simulink model "SF045A_HwAgSysArbn"  (R2013b)
settings: Solver=FixedStepDiscrete  SolverMode=SingleTasking  StartTime=0.0  StopTime=1  FixedStep=.002  RelTol=1e-3
values from neighbouring files (symbols this model uses):
  ARCHGLBPRM_2MILLISEC_SEC_F32 = DataDict.Constant    [SF045A_HwAgSysArbn_DataDict.m]
  ARCHGLBPRM_FLOATZEROTHD_ULS_F32 = DataDict.Constant    [SF045A_HwAgSysArbn_DataDict.m]
  ARCHGLBPRM_PIOVER180_ULS_F32 = DataDict.Constant    [SF045A_HwAgSysArbn_DataDict.m]
  CNVSECTOCNT_ULS_U32 = DataDict.Constant    [SF045A_HwAgSysArbn_DataDict.m]
  CNVTOMILLISEC_MILLISECPERCNT_F32 = DataDict.Constant    [SF045A_HwAgSysArbn_DataDict.m]
  FltInj_f32 = DataDict.Client    [SF045A_HwAgSysArbn_DataDict.m]
  FLTINJ_HWAGSYSARBN_HWAG = DataDict.Constant    [SF045A_HwAgSysArbn_DataDict.m]
  FLTINJ_HWAGSYSARBN_SERLCOMHWAG = DataDict.Constant    [SF045A_HwAgSysArbn_DataDict.m]
  HwAgCorrlnFlt = DataDict.NTC    [SF045A_HwAgSysArbn_DataDict.m]
  HwAgSnsrlsThdExcdd = DataDict.NTC    [SF045A_HwAgSysArbn_DataDict.m]
  HwAgSysArbnHwAgConf1Snsr = DataDict.Calibration    [SF045A_HwAgSysArbn_DataDict.m]
  HwAgSysArbnHwAgConf2Snsr = DataDict.Calibration    [SF045A_HwAgSysArbn_DataDict.m]
  HwAgSysArbnHwAgConfNoSnsr = DataDict.Calibration    [SF045A_HwAgSysArbn_DataDict.m]
  HwAgSysArbnHwAgCorrdCorrlnThd = DataDict.Calibration    [SF045A_HwAgSysArbn_DataDict.m]
  HwAgSysArbnHwAgCorrlnFailDebStep = DataDict.Calibration    [SF045A_HwAgSysArbn_DataDict.m]
  HwAgSysArbnHwAgCorrlnPassDebStep = DataDict.Calibration    [SF045A_HwAgSysArbn_DataDict.m]
  HwAgSysArbnHwAgCorrlnRng = DataDict.Calibration    [SF045A_HwAgSysArbn_DataDict.m]
  HwAgSysArbnHwAgSlewRate = DataDict.Calibration    [SF045A_HwAgSysArbn_DataDict.m]
  HwAgSysArbnHwAgSnsrlsCorrlnThd = DataDict.Calibration    [SF045A_HwAgSysArbn_DataDict.m]
  HwAgSysArbnHwAgSnsrlsKineThd = DataDict.Calibration    [SF045A_HwAgSysArbn_DataDict.m]
  HwAgSysArbnHwAgToMotAgCorrlnElpdTiLim = DataDict.Calibration    [SF045A_HwAgSysArbn_DataDict.m]
  HwAgSysArbnSerlComHwAgCorrdConf = DataDict.Calibration    [SF045A_HwAgSysArbn_DataDict.m]
  HwAgSysArbnSerlComHwAgSnsrlsConf = DataDict.Calibration    [SF045A_HwAgSysArbn_DataDict.m]
  HwAgSysArbnSlewRateTmr = DataDict.Calibration    [SF045A_HwAgSysArbn_DataDict.m]
  HWAGTHD_ULS_FLOAT32 = DataDict.Constant    [SF045A_HwAgSysArbn_DataDict.m]
  INVLDSRC_CNT_S08 = DataDict.Constant    [SF045A_HwAgSysArbn_DataDict.m]
  LRGSLEW_HWDEGPERSEC_F32 = DataDict.Constant    [SF045A_HwAgSysArbn_DataDict.m]
  NODEBSTEP_CNT_U16 = DataDict.Constant    [SF045A_HwAgSysArbn_DataDict.m]
  SLEWINPROGS_CNT_LGC = DataDict.Constant    [SF045A_HwAgSysArbn_DataDict.m]
  SLEWNOTINPROGS_CNT_LGC = DataDict.Constant    [SF045A_HwAgSysArbn_DataDict.m]
  SNSRDATASRCSELD_CNT_S08 = DataDict.Constant    [SF045A_HwAgSysArbn_DataDict.m]
  SNSRLSDATASRCSELD_CNT_S08 = DataDict.Constant    [SF045A_HwAgSysArbn_DataDict.m]
  SysGlbPrmSysKineRat = DataDict.ImprtdCal    [SF045A_HwAgSysArbn_DataDict.m]
  SysGlbPrmTorsBarStfn = DataDict.ImprtdCal    [SF045A_HwAgSysArbn_DataDict.m]
  ZEROTMR_MILLISEC_F32 = DataDict.Constant    [SF045A_HwAgSysArbn_DataDict.m]
undefined symbols (not defined in the file or in its folder): NtcSts1
libraries: NxtrLim x11, simulink x6, NxtrAbslt x6, Fil x3, autosarlib x2
(part 2 of 6)

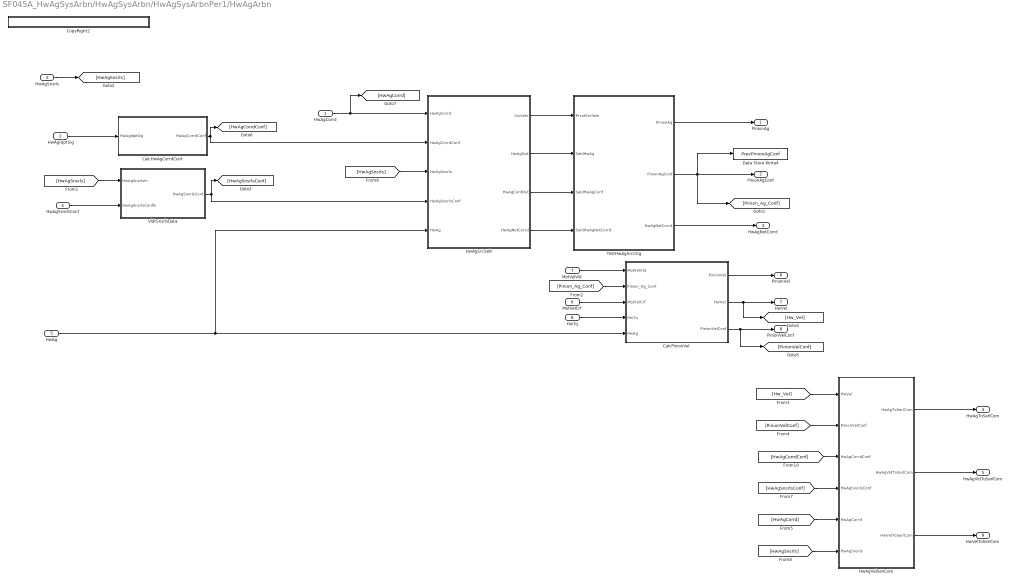
== system SF045A_HwAgSysArbn/HwAgSysArbn/HwAgSysArbnPer1/HwAgArbn ==
  HwAgCorrd : Inport
  HwAgIdptSig : Inport  Port=2
  HwAgSnsrls : Inport  Port=3
  HwAgSnsrlsConf : Inport  Port=4
  HwAg : Inport  Port=5
  MotVelCrf : Inport  Port=6
  MotVelVld : Inport  Port=7
  HwTq : Inport  Port=8
  "CalcHwAgCorrdConf " : Subsystem  RequirementInfo="{'linktype_rmi_doors' '00012ce0 (/E-STEER Core/SubSystem Specifications/Application Functions - EA4/SF045A Handwheel Angle System Arbitration)' '#SF045A_68' 'true' 'REQ:  SF045A_68' '' } %GIDa_6372da7c_5ece_4f0a_8ac6_d737184b35a8"
  CalcPinionVel : Subsystem  RequirementInfo="{'linktype_rmi_doors' '00012ce0 (/E-STEER Core/SubSystem Specifications/Application Functions - EA4/SF045A Handwheel Angle System Arbitration)' '#SF045A_138' 'true' 'REQ:  SF045A_138' '' ; 'linktype_rmi_doors' '00012ce0 (/E-STEER Core/SubSystem Specifications/Application Functions - EA4/SF045A Handwheel Angle System Arbitration)' '#SF045A_139' 'true' 'REQ:  SF045A_139' '' ; 'linktype_rmi_doors' '00012ce0 (/E-STEER Core/SubSystem Specifications/Application Functions - EA4/SF045A Handwheel Angle System Arbitration)' '#SF045A_140' 'true' 'REQ:  SF045A_140' '' ; 'linktype_rmi_doors' '00012ce0 (/E-STEER Core/SubSystem Specifications/Application Functions - EA4/SF045A Handwheel Angle System Arbitration)' '#SF045A_137' 'true' 'REQ:  SF045A_137' '' } %GIDa_9cefdf0b_14fb_482a_9d83_2c4a3ede8765"
  CopyRight2 : Subsystem  Description=|  mask(Copyright Information){none=on}
      | Copyright info block.                                               
      |                                                                     
      | Place copyright information at the top of every subsystem in design.
      mask prompts: none "No parameters"
      mask help: Place copyright information at the top of every subsystem in design.
      mask Display:
      | NxtrConf = 'Nexteer Confidential';
      | 
      | sys = bdroot; %handle for the current model ("system")
      | first = get_param(sys,'Created');
      | first = first(end-3:end);  %year is last four digits
      | 
      | last = get_param(sys,'LastModifiedDate');
      | if isempty(last)
      |     last = datestr(now,'yyyy');
      | else
      |     last = last(end-3:end);
      | end
      | 
      | if strcmp(first,last)
      |     fprintf('%s -- Copyright %s Nexteer',NxtrConf,first)
      | else
      |     fprintf('%s -- %s%s- %s Nexteer',NxtrConf,char(169),first,last)
      | end
  Data Store Write4 : DataStoreWrite  RequirementInfo={} %GIDa_c1ebf7a9_2516_4ce7_952f_4fdc50b92ec1  DataStoreName=PrevPinionAgConf
  HwAgSrcSeln : Subsystem  RequirementInfo="{'linktype_rmi_doors' '00012ce0 (/E-STEER Core/SubSystem Specifications/Application Functions - EA4/SF045A Handwheel Angle System Arbitration)' '#SF045A_71' 'true' 'REQ:  SF045A_71' '' } %GIDa_ddb011fd_98f7_44d7_8620_c4b3bd53cfc5"
  HwAgVelSeriCom : Subsystem  RequirementInfo="{'linktype_rmi_doors' '00012ce0 (/E-STEER Core/SubSystem Specifications/Application Functions - EA4/SF045A Handwheel Angle System Arbitration)' '#SF045A_85' 'true' 'REQ:  SF045A_85' '' ; 'linktype_rmi_doors' '00012ce0 (/E-STEER Core/SubSystem Specifications/Application Functions - EA4/SF045A Handwheel Angle System Arbitration)' '#SF045A_86' 'true' 'REQ:  SF045A_86' '' ; 'linktype_rmi_doors' '00012ce0 (/E-STEER Core/SubSystem Specifications/Application Functions - EA4/SF045A Handwheel Angle System Arbitration)' '#SF045A_141' 'true' 'REQ:  SF045A_141' '' ; 'linktype_rmi_doors' '00012ce0 (/E-STEER Core/SubSystem Specifications/Application Functions - EA4/SF045A Handwheel Angle System Arbitration)' '#SF045A_90' 'true' 'REQ:  SF045A_90' '' ; 'linktype_rmi_doors' '00012ce0 (/E-STEER Core/SubSystem Specifications/Application Functions - EA4/SF045A Handwheel Angle System Arbitration)' '#SF045A_87' 'true' 'REQ:  SF045A_87' '' ; 'linktype_rmi_doors' '00012ce0 (/E-STEER Core/SubSystem Specifications/Application Functions - EA4/SF045A Handwheel Angle System Arbitration)' '#SF045A_126' 'true' 'REQ:  SF045A_126' '' ; 'linktype_rmi_doors' '00012ce0 (/E-STEER Core/SubSystem Specifications/Application Functions - EA4/SF045A Handwheel Angle System Arbitration)' '#SF045A_124' 'true' 'REQ:  SF045A_124' '' ; 'linktype_rmi_doors' '00012ce0 (/E-STEER Core/SubSystem Specifications/Application Functions - EA4/SF045A Handwheel Angle System Arbitration)' '#SF045A_88' 'true' 'REQ:  SF045A_88' '' } %GIDa_7881f2ec_efdf_43f2_b299_16eeb03e4f64"
  TestHwAgSrcChg : Subsystem
  VldtSnsrlsData : Subsystem  RequirementInfo="{'linktype_rmi_doors' '00012ce0 (/E-STEER Core/SubSystem Specifications/Application Functions - EA4/SF045A Handwheel Angle System Arbitration)' '#SF045A_69' 'true' 'REQ:  SF045A_69' '' } %GIDa_369b4bc0_9330_46ed_81c8_e018ed0a07fe"
  PinionAg : Outport
  PinionAgConf : Outport  Port=2
  HwAgNotCorrd : Outport  Port=3
  HwAgToSerlCom : Outport  Port=4
  HwAgVldToSerlCom : Outport  Port=5
  PinionVel : Outport  Port=6
  HwVel : Outport  Port=7
  PinionVelConf : Outport  Port=8
  HwVelToSerlCom : Outport  Port=9
  wires:
  HwAgSrcSeln/1(SrcSeln) -> TestHwAgSrcChg/1(PrsntSrcSeln)
  HwAgSrcSeln/2(HwAgOut) -> TestHwAgSrcChg/2(SeldHwAg)
  HwAgSrcSeln/3(HwAgConfOut) -> TestHwAgSrcChg/3(SeldHwAgConf)
  HwAgSrcSeln/4(HwAgNotCorrd) -> TestHwAgSrcChg/4(SeldHwAgNotCorrd)
  TestHwAgSrcChg/1(PinionAg) -> PinionAg/1
  TestHwAgSrcChg/3(HwAgNotCorrd) -> HwAgNotCorrd/1
  [HwAgSnsrls] -> HwAgSrcSeln/3(HwAgSnsrls)
  HwAgSnsrlsConf/1 -> VldtSnsrlsData/2(HwAgSnsrlsConfIn)
  HwAgSnsrls/1 -> [HwAgSnsrls]
  HwAgCorrd/1 -> [HwAgCorrd], HwAgSrcSeln/1(HwAgCorrd)
  VldtSnsrlsData/1(HwAgSnsrlsConf) -> [HwAgSnsrlsConf], HwAgSrcSeln/4(HwAgSnsrlsConf)
  HwAgIdptSig/1 -> "CalcHwAgCorrdConf "/1(HwAgIdptSig)
  "CalcHwAgCorrdConf "/1(HwAgCorrdConf) -> [HwAgCorrdConf], HwAgSrcSeln/2(HwAgCorrdConf)
  HwAgVelSeriCom/1(HwAgToSerlCom) -> HwAgToSerlCom/1
  HwAgVelSeriCom/2(HwAgVldToSerlCom) -> HwAgVldToSerlCom/1
  [HwAgSnsrls] -> VldtSnsrlsData/1(HwAgSnsrlsIn)
  TestHwAgSrcChg/2(PinionAgConf) -> Data Store Write4/1, [Pinion_Ag_Conf], PinionAgConf/1
  MotVelCrf/1 -> CalcPinionVel/3(MotVelCrf)
  MotVelVld/1 -> CalcPinionVel/1(MotVelVld)
  HwTq/1 -> CalcPinionVel/4(HwTq)
  CalcPinionVel/1(PinionVel) -> PinionVel/1
  CalcPinionVel/2(HwVel) -> [Hw_Vel], HwVel/1
  CalcPinionVel/3(PinionVelConf) -> [PinionVelConf], PinionVelConf/1
  HwAg/1 -> HwAgSrcSeln/5(HwAg), CalcPinionVel/5(HwAg)
  HwAgVelSeriCom/3(HwVelToSerlCom) -> HwVelToSerlCom/1
  [Hw_Vel] -> HwAgVelSeriCom/1(HwVel)
  [PinionVelConf] -> HwAgVelSeriCom/2(PinionVelConf)
  [HwAgCorrdConf] -> HwAgVelSeriCom/3(HwAgCorrdConf)
  [HwAgSnsrlsConf] -> HwAgVelSeriCom/4(HwAgSnsrlsConf)
  [Pinion_Ag_Conf] -> CalcPinionVel/2(Pinion_Ag_Conf)
  [HwAgCorrd] -> HwAgVelSeriCom/5(HwAgCorrd)
  [HwAgSnsrls] -> HwAgVelSeriCom/6(HwAgSnsrls)

== system SF045A_HwAgSysArbn/HwAgSysArbn/HwAgSysArbnInit1/GetRefTmr100MicroSec32bit/CopyRight2 ==

== system SF045A_HwAgSysArbn/HwAgSysArbn/HwAgSysArbnInit1/Kinematic Integrity/SetNtcSts ==
  note: Note:
      |
      | - "ISO Fault Debounce Design" Simulink block intent to use here for Simulation purpose only. Do not Code this block
  NtcNr : Inport
  NtcStInfo : Inport  Port=2
  NtcSts : Inport  Port=3
  DebStep : Inport  Port=4
  CopyRight2 : Subsystem  Description=|  mask(Copyright Information){none=on}
      | Copyright info block.                                               
      |                                                                     
      | Place copyright information at the top of every subsystem in design.
      mask prompts: none "No parameters"
      mask help: Place copyright information at the top of every subsystem in design.
      mask Display:
      | NxtrConf = 'Nexteer Confidential';
      | 
      | sys = bdroot; %handle for the current model ("system")
      | first = get_param(sys,'Created');
      | if(isempty(first))
      |     first = datestr(now,'yyyy');
      | else
      |     first = first(end-3:end);  %year is last four digits
      | end
      | 
      | last = get_param(sys,'LastModifiedDate');
      | if isempty(last)
      |     last = datestr(now,'yyyy');
      | else
      |     last = last(end-3:end);
      | end
      | 
      | if strcmp(first,last)
      |     fprintf('%s -- Copyright %s Nexteer',NxtrConf,first)
      | else
      |     fprintf('%s -- %s%s- %s Nexteer',NxtrConf,char(169),first,last)
      | end
  Data Store Write : DataStoreWrite  DataStoreName=NtcQlfr
  Data Store Write1 : DataStoreWrite  DataStoreName=NtcQlfrHwAgSnsrlsThdExcd
  Data Store Write2 : DataStoreWrite  DataStoreName=NtcStInfoHwAgSnsrlsThdExcd
  Data Store Write3 : DataStoreWrite  DataStoreName=NtcStsHwAgSnsrlsThdExcd
  Data Type Conversion : DataTypeConversion  OutDataTypeStr=Enum: SigQlfr1
  Data Type Conversion1 : DataTypeConversion  OutDataTypeStr=uint8
  Ground : Ground
  ISO Fault Debounce Design : Stateflow chart  TreatAsAtomicUnit=on
      settings: AttributesFormatString=|
      | Simulation Purpose Only.
      | Do Not Code this block
      | Diagnostic Manager Owns this requirement
  Terminator : Terminator
  Terminator1 : Terminator
  wires:
  Data Type Conversion1/1 -> Data Store Write2/1
  NtcStInfo/1 -> Terminator1/1, Data Type Conversion1/1
  NtcSts/1 -> ISO Fault Debounce Design/1(NtcSts), Data Store Write3/1
  Data Type Conversion/1 -> Data Store Write/1, Data Store Write1/1
  Ground/1 -> ISO Fault Debounce Design/3(SvcClr)
  ISO Fault Debounce Design/1(Qualifier) -> Data Type Conversion/1
  DebStep/1 -> ISO Fault Debounce Design/2(DebStep)
  NtcNr/1 -> Terminator/1

== system SF045A_HwAgSysArbn/HwAgSysArbn/HwAgSysArbnPer1/FltInj_f32 client/CodeGen ==
  note: FltInj_f32(float32 *SigPah, uint16 LocnKey)
  note: NOTE 1:  Simulink 2013b cannot handle InOut arguments, so the operation
      |                 prototype inside this block is not quite right.
      |
      | NOTE 2:  Do not use this variant for simulation.  Sig_Out = zero, always.
  Sig : Inport
  "LocnKey  " : Inport  Port=2
  CopyRight1 : Subsystem  Description=|  mask(Copyright Information){none=on}
      | Copyright info block.                                               
      |                                                                     
      | Place copyright information at the top of every subsystem in design.
      mask prompts: none "No parameters"
      mask help: Place copyright information at the top of every subsystem in design.
      mask Display:
      | NxtrConf = 'Nexteer Confidential';
      | 
      | sys = bdroot; %handle for the current model ("system")
      | first = get_param(sys,'Created');
      | if(isempty(first))
      |     first = datestr(now,'yyyy');
      | else
      |     first = first(end-3:end);  %year is last four digits
      | end
      | 
      | last = get_param(sys,'LastModifiedDate');
      | if isempty(last)
      |     last = datestr(now,'yyyy');
      | else
      |     last = last(end-3:end);
      | end
      | 
      | if strcmp(first,last)
      |     fprintf('%s -- Copyright %s Nexteer',NxtrConf,first)
      | else
      |     fprintf('%s -- %s%s- %s Nexteer',NxtrConf,char(169),first,last)
      | end
  Invoke AUTOSAR Server Operation : autosarlib/Invoke AUTOSAR Server Operation  portName=FltInj_f32  operationPrototype=FltInj_f32(IN single SigPah_ArgIn, OUT single SigPah_ArgOut, IN uint16 LocnKey)  interfacePath=/AUTOSAR/Interface  serverType=Application software  showErrorStatus=off  SAMPLETIME=-1  showARPortLabels=on
  Sig_Out : Outport  OutDataTypeStr=single
  wires:
  Invoke AUTOSAR Server Operation/1 -> Sig_Out/1
  "LocnKey  "/1 -> Invoke AUTOSAR Server Operation/2
  Sig/1 -> Invoke AUTOSAR Server Operation/1

== system SF045A_HwAgSysArbn/HwAgSysArbn/HwAgSysArbnPer1/FltInj_f32 client/CopyRight1 ==

== system SF045A_HwAgSysArbn/HwAgSysArbn/HwAgSysArbnPer1/FltInj_f32 client/CopyRight2 ==

== system SF045A_HwAgSysArbn/HwAgSysArbn/HwAgSysArbnPer1/FltInj_f32 client/Sim ==
  note: EA4.x Fault Injection
  note: This block requires no modification by FDD author.
      |
      | This block does not actually simulate any fault injection.  It is simply a pass-thru.
      |
      | Input port (#2) simply terminates its signal, but we are trying to force the FDD author
      | to properly use the FltInjectionLocType enumeration in FDD model.
  Sig : Inport
  "LocnKey  " : Inport  Port=2  OutDataTypeStr=uint16
  CopyRight1 : Subsystem  Description=|  mask(Copyright Information){none=on}
      | Copyright info block.                                               
      |                                                                     
      | Place copyright information at the top of every subsystem in design.
      mask prompts: none "No parameters"
      mask help: Place copyright information at the top of every subsystem in design.
      mask Display:
      | NxtrConf = 'Nexteer Confidential';
      | 
      | sys = bdroot; %handle for the current model ("system")
      | first = get_param(sys,'Created');
      | if(isempty(first))
      |     first = datestr(now,'yyyy');
      | else
      |     first = first(end-3:end);  %year is last four digits
      | end
      | 
      | last = get_param(sys,'LastModifiedDate');
      | if isempty(last)
      |     last = datestr(now,'yyyy');
      | else
      |     last = last(end-3:end);
      | end
      | 
      | if strcmp(first,last)
      |     fprintf('%s -- Copyright %s Nexteer',NxtrConf,first)
      | else
      |     fprintf('%s -- %s%s- %s Nexteer',NxtrConf,char(169),first,last)
      | end
  Terminator : Terminator
  Sig_Out : Outport
  wires:
  "LocnKey  "/1 -> Terminator/1
  Sig/1 -> Sig_Out/1

== system SF045A_HwAgSysArbn/HwAgSysArbn/HwAgSysArbnPer1/FltInj_f32 client1/CodeGen ==
  note: NOTE 1:  Simulink 2013b cannot handle InOut arguments, so the operation
      |                 prototype inside this block is not quite right.
      |
      | NOTE 2:  Do not use this variant for simulation.  Sig_Out = zero, always.
  note: FltInj_f32(float32 *SigPah, uint16 LocnKey)
  Sig : Inport
  "LocnKey  " : Inport  Port=2
  CopyRight1 : Subsystem  Description=|  mask(Copyright Information){none=on}
      | Copyright info block.                                               
      |                                                                     
      | Place copyright information at the top of every subsystem in design.
      mask prompts: none "No parameters"
      mask help: Place copyright information at the top of every subsystem in design.
      mask Display:
      | NxtrConf = 'Nexteer Confidential';
      | 
      | sys = bdroot; %handle for the current model ("system")
      | first = get_param(sys,'Created');
      | if(isempty(first))
      |     first = datestr(now,'yyyy');
      | else
      |     first = first(end-3:end);  %year is last four digits
      | end
      | 
      | last = get_param(sys,'LastModifiedDate');
      | if isempty(last)
      |     last = datestr(now,'yyyy');
      | else
      |     last = last(end-3:end);
      | end
      | 
      | if strcmp(first,last)
      |     fprintf('%s -- Copyright %s Nexteer',NxtrConf,first)
      | else
      |     fprintf('%s -- %s%s- %s Nexteer',NxtrConf,char(169),first,last)
      | end
  Invoke AUTOSAR Server Operation : autosarlib/Invoke AUTOSAR Server Operation  portName=FltInj_f32  operationPrototype=FltInj_f32(IN single SigPah_ArgIn, OUT single SigPah_ArgOut, IN uint16 LocnKey)  interfacePath=/AUTOSAR/Interface  serverType=Application software  showErrorStatus=off  SAMPLETIME=-1  showARPortLabels=on
  Sig_Out : Outport  OutDataTypeStr=single
  wires:
  Sig/1 -> Invoke AUTOSAR Server Operation/1
  "LocnKey  "/1 -> Invoke AUTOSAR Server Operation/2
  Invoke AUTOSAR Server Operation/1 -> Sig_Out/1

== system SF045A_HwAgSysArbn/HwAgSysArbn/HwAgSysArbnPer1/FltInj_f32 client1/CopyRight1 ==

== system SF045A_HwAgSysArbn/HwAgSysArbn/HwAgSysArbnPer1/FltInj_f32 client1/CopyRight2 ==

== system SF045A_HwAgSysArbn/HwAgSysArbn/HwAgSysArbnPer1/FltInj_f32 client1/Sim ==
  note: This block requires no modification by FDD author.
      |
      | This block does not actually simulate any fault injection.  It is simply a pass-thru.
      |
      | Input port (#2) simply terminates its signal, but we are trying to force the FDD author
      | to properly use the FltInjectionLocType enumeration in FDD model.
  note: EA4.x Fault Injection
  Sig : Inport
  "LocnKey  " : Inport  Port=2  OutDataTypeStr=uint16
  CopyRight1 : Subsystem  Description=|  mask(Copyright Information){none=on}
      | Copyright info block.                                               
      |                                                                     
      | Place copyright information at the top of every subsystem in design.
      mask prompts: none "No parameters"
      mask help: Place copyright information at the top of every subsystem in design.
      mask Display:
      | NxtrConf = 'Nexteer Confidential';
      | 
      | sys = bdroot; %handle for the current model ("system")
      | first = get_param(sys,'Created');
      | if(isempty(first))
      |     first = datestr(now,'yyyy');
      | else
      |     first = first(end-3:end);  %year is last four digits
      | end
      | 
      | last = get_param(sys,'LastModifiedDate');
      | if isempty(last)
      |     last = datestr(now,'yyyy');
      | else
      |     last = last(end-3:end);
      | end
      | 
      | if strcmp(first,last)
      |     fprintf('%s -- Copyright %s Nexteer',NxtrConf,first)
      | else
      |     fprintf('%s -- %s%s- %s Nexteer',NxtrConf,char(169),first,last)
      | end
  Terminator : Terminator
  Sig_Out : Outport
  wires:
  Sig/1 -> Sig_Out/1
  "LocnKey  "/1 -> Terminator/1

== system SF045A_HwAgSysArbn/HwAgSysArbn/HwAgSysArbnPer1/HwAgArbn/CalcHwAgCorrdConf  ==
  HwAgIdptSig : Inport
  CopyRight2 : Subsystem  Description=|  mask(Copyright Information){none=on}
      | Copyright info block.                                               
      |                                                                     
      | Place copyright information at the top of every subsystem in design.
      mask prompts: none "No parameters"
      mask help: Place copyright information at the top of every subsystem in design.
      mask Display:
      | NxtrConf = 'Nexteer Confidential';
      | 
      | sys = bdroot; %handle for the current model ("system")
      | first = get_param(sys,'Created');
      | first = first(end-3:end);  %year is last four digits
      | 
      | last = get_param(sys,'LastModifiedDate');
      | if isempty(last)
      |     last = datestr(now,'yyyy');
      | else
      |     last = last(end-3:end);
      | end
      | 
      | if strcmp(first,last)
      |     fprintf('%s -- Copyright %s Nexteer',NxtrConf,first)
      | else
      |     fprintf('%s -- %s%s- %s Nexteer',NxtrConf,char(169),first,last)
      | end
  Merge1 : Merge  RequirementInfo="{'linktype_rmi_doors' '00012ce0 (/E-STEER Core/SubSystem Specifications/Application Functions - EA4/SF045A Handwheel Angle System Arbitration)' '#SF045A_68' 'true' 'REQ:  SF045A_68' '' } %GIDa_8ba7271c_3c6f_4c09_8c6a_0996d4bd89c4"  Inputs=4
  NoSensor : Subsystem  RequirementInfo="{'linktype_rmi_doors' '00012ce0 (/E-STEER Core/SubSystem Specifications/Application Functions - EA4/SF045A Handwheel Angle System Arbitration)' '#SF045A_68' 'true' 'REQ:  SF045A_68' '' } %GIDa_bcddfe72_8a7a_46d1_a6ba_ba8d8ba7ffeb"  TreatAsAtomicUnit=on
  OneSensor : Subsystem  RequirementInfo="{'linktype_rmi_doors' '00012ce0 (/E-STEER Core/SubSystem Specifications/Application Functions - EA4/SF045A Handwheel Angle System Arbitration)' '#SF045A_68' 'true' 'REQ:  SF045A_68' '' } %GIDa_0a3dc2be_c596_4c40_aca6_3757520fa4fc"  TreatAsAtomicUnit=on
  Switch Case : SwitchCase  CaseConditions={0,1,2}
  TwoSensors : Subsystem  RequirementInfo="{'linktype_rmi_doors' '00012ce0 (/E-STEER Core/SubSystem Specifications/Application Functions - EA4/SF045A Handwheel Angle System Arbitration)' '#SF045A_68' 'true' 'REQ:  SF045A_68' '' } %GIDa_53776eb7_3fdf_44ee_86de_ad7f9ec7a3c3"  TreatAsAtomicUnit=on
  Zero : Subsystem  RequirementInfo="{'linktype_rmi_doors' '00012ce0 (/E-STEER Core/SubSystem Specifications/Application Functions - EA4/SF045A Handwheel Angle System Arbitration)' '#SF045A_68' 'true' 'REQ:  SF045A_68' '' } %GIDa_3c71ffef_8e48_445f_a345_c5683038ce66"  TreatAsAtomicUnit=on
  HwAgCorrdConf : Outport
  wires:
  HwAgIdptSig/1 -> Switch Case/1
  Switch Case/1 -> NoSensor/Action
  Switch Case/4 -> Zero/Action
  Merge1/1 -> HwAgCorrdConf/1
  Switch Case/3 -> TwoSensors/Action
  Switch Case/2 -> OneSensor/Action
  NoSensor/1(Out1) -> Merge1/1
  OneSensor/1(Out1) -> Merge1/2
  TwoSensors/1(Out1) -> Merge1/3
  Zero/1(Out1) -> Merge1/4

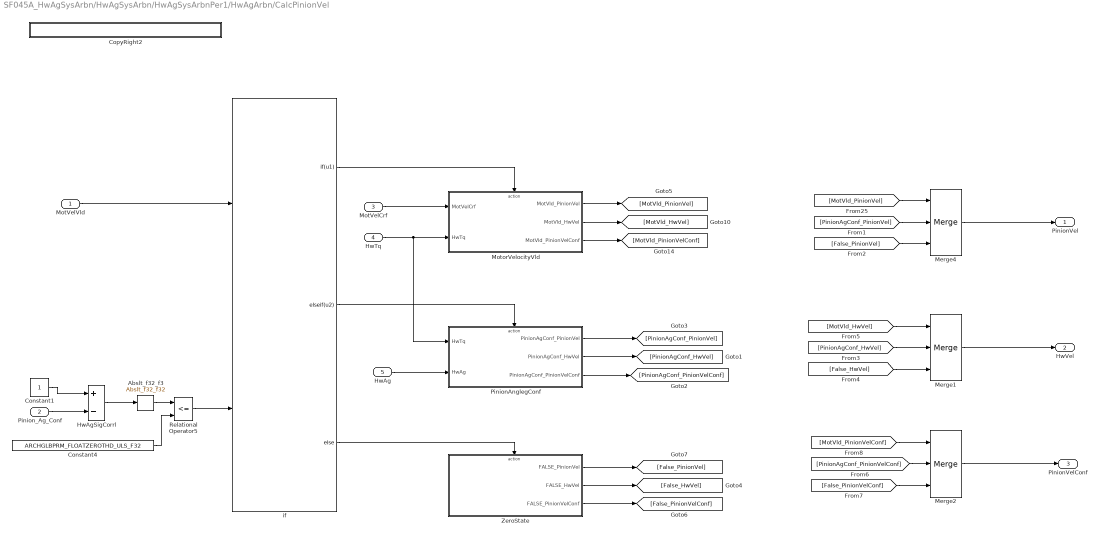
== system SF045A_HwAgSysArbn/HwAgSysArbn/HwAgSysArbnPer1/HwAgArbn/CalcPinionVel ==
  MotVelVld : Inport
  Pinion_Ag_Conf : Inport  Port=2
  MotVelCrf : Inport  Port=3
  HwTq : Inport  Port=4
  HwAg : Inport  Port=5
  Abslt_f32_f3 : NxtrAbslt/Abslt_f32_f32  RequirementInfo={} %GIDa_6df87594_202b_42cc_b14d_962ac3ebd229  SFunctionSpec=single y1 = Abslt_f32_f32(single u1)
      settings: AttributesFormatString=%<Name>
  Constant1 : Constant  OutDataTypeStr=single
      settings: AttributesFormatString=%<OutDataTypeStr>
  Constant4 : Constant  RequirementInfo={} %GIDa_34a287e4_a6a8_4918_832c_301bf2b35dc4  Value=ARCHGLBPRM_FLOATZEROTHD_ULS_F32
  CopyRight2 : Subsystem  Description=|  mask(Copyright Information){none=on}
      | Copyright info block.                                               
      |                                                                     
      | Place copyright information at the top of every subsystem in design.
      mask prompts: none "No parameters"
      mask help: Place copyright information at the top of every subsystem in design.
      mask Display:
      | NxtrConf = 'Nexteer Confidential';
      | 
      | sys = bdroot; %handle for the current model ("system")
      | first = get_param(sys,'Created');
      | first = first(end-3:end);  %year is last four digits
      | 
      | last = get_param(sys,'LastModifiedDate');
      | if isempty(last)
      |     last = datestr(now,'yyyy');
      | else
      |     last = last(end-3:end);
      | end
      | 
      | if strcmp(first,last)
      |     fprintf('%s -- Copyright %s Nexteer',NxtrConf,first)
      | else
      |     fprintf('%s -- %s%s- %s Nexteer',NxtrConf,char(169),first,last)
      | end
  HwAgSigCorrl : Sum  RequirementInfo="{'linktype_rmi_doors' '00012ce0 (/E-STEER Core/SubSystem Specifications/Application Functions - EA4/SF045A Handwheel Angle System Arbitration)' '#SF045A_105' 'true' 'REQ:  SF045A_105' '' } %GIDa_95324c42_1f33_414b_9524_4a8136d78cff"  Inputs=+-
  Merge1 : Merge  RequirementInfo="{'linktype_rmi_doors' '00012ce0 (/E-STEER Core/SubSystem Specifications/Application Functions - EA4/SF045A Handwheel Angle System Arbitration)' '#SF045A_138' 'true' 'REQ:  SF045A_138' '' ; 'linktype_rmi_doors' '00012ce0 (/E-STEER Core/SubSystem Specifications/Application Functions - EA4/SF045A Handwheel Angle System Arbitration)' '#SF045A_139' 'true' 'REQ:  SF045A_139' '' ; 'linktype_rmi_doors' '00012ce0 (/E-STEER Core/SubSystem Specifications/Application Functions - EA4/SF045A Handwheel Angle System Arbitration)' '#SF045A_140' 'true' 'REQ:  SF045A_140' '' } %GIDa_f50f6f0b_7fa2_46d1_ac72_1e122ca2c0fd"  Inputs=3
  Merge2 : Merge  RequirementInfo="{'linktype_rmi_doors' '00012ce0 (/E-STEER Core/SubSystem Specifications/Application Functions - EA4/SF045A Handwheel Angle System Arbitration)' '#SF045A_138' 'true' 'REQ:  SF045A_138' '' ; 'linktype_rmi_doors' '00012ce0 (/E-STEER Core/SubSystem Specifications/Application Functions - EA4/SF045A Handwheel Angle System Arbitration)' '#SF045A_139' 'true' 'REQ:  SF045A_139' '' ; 'linktype_rmi_doors' '00012ce0 (/E-STEER Core/SubSystem Specifications/Application Functions - EA4/SF045A Handwheel Angle System Arbitration)' '#SF045A_140' 'true' 'REQ:  SF045A_140' '' } %GIDa_67d2558a_e011_4990_9602_7b20b170760f"  Inputs=3
  Merge4 : Merge  RequirementInfo="{'linktype_rmi_doors' '00012ce0 (/E-STEER Core/SubSystem Specifications/Application Functions - EA4/SF045A Handwheel Angle System Arbitration)' '#SF045A_140' 'true' 'REQ:  SF045A_140' '' ; 'linktype_rmi_doors' '00012ce0 (/E-STEER Core/SubSystem Specifications/Application Functions - EA4/SF045A Handwheel Angle System Arbitration)' '#SF045A_138' 'true' 'REQ:  SF045A_138' '' ; 'linktype_rmi_doors' '00012ce0 (/E-STEER Core/SubSystem Specifications/Application Functions - EA4/SF045A Handwheel Angle System Arbitration)' '#SF045A_139' 'true' 'REQ:  SF045A_139' '' } %GIDa_518bee00_1bab_4dbe_9172_b7efbfa1d3a2"  Inputs=3
  MotorVelocityVld : Subsystem  RequirementInfo="{'linktype_rmi_doors' '00012ce0 (/E-STEER Core/SubSystem Specifications/Application Functions - EA4/SF045A Handwheel Angle System Arbitration)' '#SF045A_137' 'true' 'REQ:  SF045A_137' '' ; 'linktype_rmi_doors' '00012ce0 (/E-STEER Core/SubSystem Specifications/Application Functions - EA4/SF045A Handwheel Angle System Arbitration)' '#SF045A_138' 'true' 'REQ:  SF045A_138' '' } %GIDa_20abc8f5_e256_40b7_83db_f3e29654aacd"  TreatAsAtomicUnit=on
  PinionAnglegConf : Subsystem  RequirementInfo="{'linktype_rmi_doors' '00012ce0 (/E-STEER Core/SubSystem Specifications/Application Functions - EA4/SF045A Handwheel Angle System Arbitration)' '#SF045A_139' 'true' 'REQ:  SF045A_139' '' } %GIDa_2372bfca_2df7_43c4_87e6_2086174cc9a0"  TreatAsAtomicUnit=on
  Relational Operator5 : RelationalOperator  RequirementInfo="{'linktype_rmi_doors' '00012ce0 (/E-STEER Core/SubSystem Specifications/Application Functions - EA4/SF045A Handwheel Angle System Arbitration)' '#SF045A_104' 'true' 'REQ:  SF045A_104' '' ; 'linktype_rmi_doors' '00012ce0 (/E-STEER Core/SubSystem Specifications/Application Functions - EA4/SF045A Handwheel Angle System Arbitration)' '#SF045A_85' 'true' 'REQ:  SF045A_85' '' } %GIDa_50f7561d_81c0_41d3_892b_68c24874fab0"  Operator=<=  OutDataTypeStr=boolean
  ZeroState : Subsystem  RequirementInfo="{'linktype_rmi_doors' '00012ce0 (/E-STEER Core/SubSystem Specifications/Application Functions - EA4/SF045A Handwheel Angle System Arbitration)' '#SF045A_140' 'true' 'REQ:  SF045A_140' '' } %GIDa_485f4ca6_bda0_4675_8768_534628d290f5"  TreatAsAtomicUnit=on
  if : If  RequirementInfo="{'linktype_rmi_doors' '00012ce0 (/E-STEER Core/SubSystem Specifications/Application Functions - EA4/SF045A Handwheel Angle System Arbitration)' '#SF045A_138' 'true' 'REQ:  SF045A_138' '' ; 'linktype_rmi_doors' '00012ce0 (/E-STEER Core/SubSystem Specifications/Application Functions - EA4/SF045A Handwheel Angle System Arbitration)' '#SF045A_140' 'true' 'REQ:  SF045A_140' '' ; 'linktype_rmi_doors' '00012ce0 (/E-STEER Core/SubSystem Specifications/Application Functions - EA4/SF045A Handwheel Angle System Arbitration)' '#SF045A_139' 'true' 'REQ:  SF045A_139' '' } %GIDa_f1e8ca97_589f_41fa_ad21_adfe6884b23f"  NumInputs=2  IfExpression=u1  ElseIfExpressions=u2
  PinionVel : Outport
  HwVel : Outport  Port=2
  PinionVelConf : Outport  Port=3
  wires:
  MotVelVld/1 -> if/1
  if/1 -> MotorVelocityVld/Action
  if/2 -> PinionAnglegConf/Action
  if/3 -> ZeroState/Action
  MotorVelocityVld/1(MotVld_PinionVel) -> [MotVld_PinionVel]
  MotorVelocityVld/2(MotVld_HwVel) -> [MotVld_HwVel]
  MotorVelocityVld/3(MotVld_PinionVelConf) -> [MotVld_PinionVelConf]
  PinionAnglegConf/1(PinionAgConf_PinionVel) -> [PinionAgConf_PinionVel]
  PinionAnglegConf/2(PinionAgConf_HwVel) -> [PinionAgConf_HwVel]
  PinionAnglegConf/3(PinionAgConf_PinionVelConf) -> [PinionAgConf_PinionVelConf]
  ZeroState/1(FALSE_PinionVel) -> [False_PinionVel]
  ZeroState/2(FALSE_HwVel) -> [False_HwVel]
  ZeroState/3(FALSE_PinionVelConf) -> [False_PinionVelConf]
  [MotVld_PinionVel] -> Merge4/1
  [PinionAgConf_PinionVel] -> Merge4/2
  [False_PinionVel] -> Merge4/3
  [MotVld_HwVel] -> Merge1/1
  [PinionAgConf_HwVel] -> Merge1/2
  [False_HwVel] -> Merge1/3
  [MotVld_PinionVelConf] -> Merge2/1
  [PinionAgConf_PinionVelConf] -> Merge2/2
  [False_PinionVelConf] -> Merge2/3
  Merge4/1 -> PinionVel/1
  Merge1/1 -> HwVel/1
  MotVelCrf/1 -> MotorVelocityVld/1(MotVelCrf)
  HwTq/1 -> PinionAnglegConf/1(HwTq), MotorVelocityVld/2(HwTq)
  HwAg/1 -> PinionAnglegConf/2(HwAg)
  Relational Operator5/1 -> if/2
  Merge2/1 -> PinionVelConf/1
  HwAgSigCorrl/1 -> Abslt_f32_f3/1
  Constant4/1 -> Relational Operator5/2
  Abslt_f32_f3/1 -> Relational Operator5/1
  Pinion_Ag_Conf/1 -> HwAgSigCorrl/2
  Constant1/1 -> HwAgSigCorrl/1

== system SF045A_HwAgSysArbn/HwAgSysArbn/HwAgSysArbnPer1/HwAgArbn/CopyRight2 ==

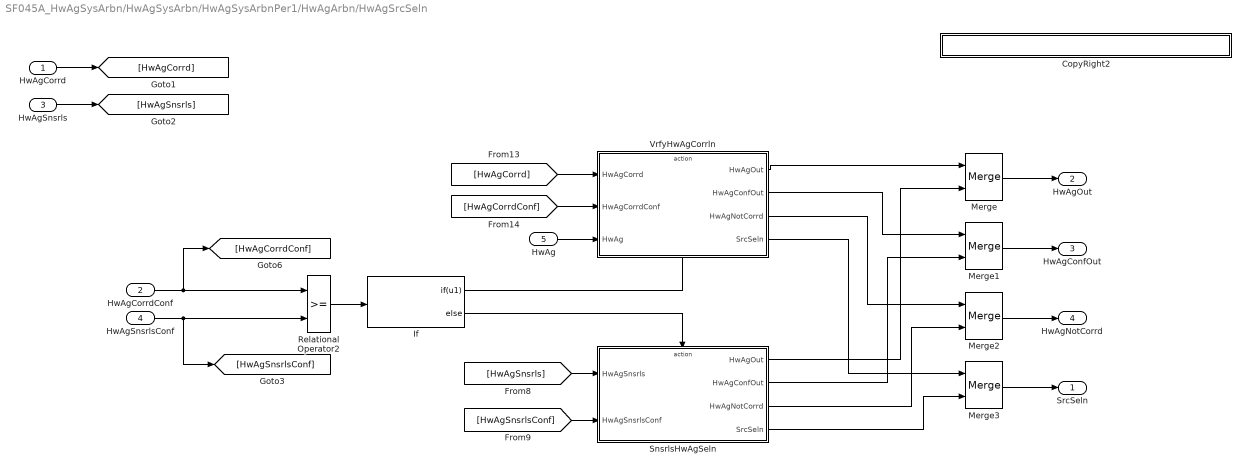
== system SF045A_HwAgSysArbn/HwAgSysArbn/HwAgSysArbnPer1/HwAgArbn/HwAgSrcSeln ==
  HwAgCorrd : Inport
  HwAgCorrdConf : Inport  Port=2
  HwAgSnsrls : Inport  Port=3
  HwAgSnsrlsConf : Inport  Port=4
  HwAg : Inport  Port=5
  CopyRight2 : Subsystem  Description=|  mask(Copyright Information){none=on}
      | Copyright info block.                                               
      |                                                                     
      | Place copyright information at the top of every subsystem in design.
      mask prompts: none "No parameters"
      mask help: Place copyright information at the top of every subsystem in design.
      mask Display:
      | NxtrConf = 'Nexteer Confidential';
      | 
      | sys = bdroot; %handle for the current model ("system")
      | first = get_param(sys,'Created');
      | first = first(end-3:end);  %year is last four digits
      | 
      | last = get_param(sys,'LastModifiedDate');
      | if isempty(last)
      |     last = datestr(now,'yyyy');
      | else
      |     last = last(end-3:end);
      | end
      | 
      | if strcmp(first,last)
      |     fprintf('%s -- Copyright %s Nexteer',NxtrConf,first)
      | else
      |     fprintf('%s -- %s%s- %s Nexteer',NxtrConf,char(169),first,last)
      | end
  If : If  RequirementInfo="{'linktype_rmi_doors' '00012ce0 (/E-STEER Core/SubSystem Specifications/Application Functions - EA4/SF045A Handwheel Angle System Arbitration)' '#SF045A_125' 'true' 'REQ:  SF045A_125' '' ; 'linktype_rmi_doors' '00012ce0 (/E-STEER Core/SubSystem Specifications/Application Functions - EA4/SF045A Handwheel Angle System Arbitration)' '#SF045A_71' 'true' 'REQ:  SF045A_71' '' ; 'linktype_rmi_doors' '00012ce0 (/E-STEER Core/SubSystem Specifications/Application Functions - EA4/SF045A Handwheel Angle System Arbitration)' '#SF045A_76' 'true' 'REQ:  SF045A_76' '' ; 'linktype_rmi_doors' '00012ce0 (/E-STEER Core/SubSystem Specifications/Application Functions - EA4/SF045A Handwheel Angle System Arbitration)' '#SF045A_73' 'true' 'REQ:  SF045A_73' '' } %GIDa_e0679fc8_1d6a_4c30_8af2_f6ddfb6a44f9"  IfExpression=u1
  Merge : Merge  RequirementInfo="{'linktype_rmi_doors' '00012ce0 (/E-STEER Core/SubSystem Specifications/Application Functions - EA4/SF045A Handwheel Angle System Arbitration)' '#SF045A_71' 'true' 'REQ:  SF045A_71' '' ; 'linktype_rmi_doors' '00012ce0 (/E-STEER Core/SubSystem Specifications/Application Functions - EA4/SF045A Handwheel Angle System Arbitration)' '#SF045A_73' 'true' 'REQ:  SF045A_73' '' ; 'linktype_rmi_doors' '00012ce0 (/E-STEER Core/SubSystem Specifications/Application Functions - EA4/SF045A Handwheel Angle System Arbitration)' '#SF045A_125' 'true' 'REQ:  SF045A_125' '' ; 'linktype_rmi_doors' '00012ce0 (/E-STEER Core/SubSystem Specifications/Application Functions - EA4/SF045A Handwheel Angle System Arbitration)' '#SF045A_76' 'true' 'REQ:  SF045A_76' '' } %GIDa_3828973d_c93b_4cf8_b002_dcf18215c546"
  Merge1 : Merge  RequirementInfo="{'linktype_rmi_doors' '00012ce0 (/E-STEER Core/SubSystem Specifications/Application Functions - EA4/SF045A Handwheel Angle System Arbitration)' '#SF045A_71' 'true' 'REQ:  SF045A_71' '' ; 'linktype_rmi_doors' '00012ce0 (/E-STEER Core/SubSystem Specifications/Application Functions - EA4/SF045A Handwheel Angle System Arbitration)' '#SF045A_73' 'true' 'REQ:  SF045A_73' '' ; 'linktype_rmi_doors' '00012ce0 (/E-STEER Core/SubSystem Specifications/Application Functions - EA4/SF045A Handwheel Angle System Arbitration)' '#SF045A_125' 'true' 'REQ:  SF045A_125' '' ; 'linktype_rmi_doors' '00012ce0 (/E-STEER Core/SubSystem Specifications/Application Functions - EA4/SF045A Handwheel Angle System Arbitration)' '#SF045A_76' 'true' 'REQ:  SF045A_76' '' } %GIDa_ca4bca52_c5a1_486a_9ac5_fae38e1d3555"
  Merge2 : Merge  RequirementInfo="{'linktype_rmi_doors' '00012ce0 (/E-STEER Core/SubSystem Specifications/Application Functions - EA4/SF045A Handwheel Angle System Arbitration)' '#SF045A_71' 'true' 'REQ:  SF045A_71' '' ; 'linktype_rmi_doors' '00012ce0 (/E-STEER Core/SubSystem Specifications/Application Functions - EA4/SF045A Handwheel Angle System Arbitration)' '#SF045A_73' 'true' 'REQ:  SF045A_73' '' ; 'linktype_rmi_doors' '00012ce0 (/E-STEER Core/SubSystem Specifications/Application Functions - EA4/SF045A Handwheel Angle System Arbitration)' '#SF045A_125' 'true' 'REQ:  SF045A_125' '' ; 'linktype_rmi_doors' '00012ce0 (/E-STEER Core/SubSystem Specifications/Application Functions - EA4/SF045A Handwheel Angle System Arbitration)' '#SF045A_76' 'true' 'REQ:  SF045A_76' '' } %GIDa_9d637fe5_8a5c_4635_ba41_06e0ea4e998a"
  Merge3 : Merge  RequirementInfo="{'linktype_rmi_doors' '00012ce0 (/E-STEER Core/SubSystem Specifications/Application Functions - EA4/SF045A Handwheel Angle System Arbitration)' '#SF045A_71' 'true' 'REQ:  SF045A_71' '' ; 'linktype_rmi_doors' '00012ce0 (/E-STEER Core/SubSystem Specifications/Application Functions - EA4/SF045A Handwheel Angle System Arbitration)' '#SF045A_73' 'true' 'REQ:  SF045A_73' '' ; 'linktype_rmi_doors' '00012ce0 (/E-STEER Core/SubSystem Specifications/Application Functions - EA4/SF045A Handwheel Angle System Arbitration)' '#SF045A_125' 'true' 'REQ:  SF045A_125' '' ; 'linktype_rmi_doors' '00012ce0 (/E-STEER Core/SubSystem Specifications/Application Functions - EA4/SF045A Handwheel Angle System Arbitration)' '#SF045A_76' 'true' 'REQ:  SF045A_76' '' } %GIDa_4e7db8e0_7a75_4463_bb70_e8d016ad650a"
  Relational Operator2 : RelationalOperator  RequirementInfo="{'linktype_rmi_doors' '00012ce0 (/E-STEER Core/SubSystem Specifications/Application Functions - EA4/SF045A Handwheel Angle System Arbitration)' '#SF045A_71' 'true' 'REQ:  SF045A_71' '' ; 'linktype_rmi_doors' '00012ce0 (/E-STEER Core/SubSystem Specifications/Application Functions - EA4/SF045A Handwheel Angle System Arbitration)' '#SF045A_125' 'true' 'REQ:  SF045A_125' '' ; 'linktype_rmi_doors' '00012ce0 (/E-STEER Core/SubSystem Specifications/Application Functions - EA4/SF045A Handwheel Angle System Arbitration)' '#SF045A_73' 'true' 'REQ:  SF045A_73' '' ; 'linktype_rmi_doors' '00012ce0 (/E-STEER Core/SubSystem Specifications/Application Functions - EA4/SF045A Handwheel Angle System Arbitration)' '#SF045A_76' 'true' 'REQ:  SF045A_76' '' } %GIDa_4bcb8f9e_c2e2_4446_aec4_326177f7fbb0"  OutDataTypeStr=boolean
  SnsrlsHwAgSeln : Subsystem  RequirementInfo="{'linktype_rmi_doors' '00012ce0 (/E-STEER Core/SubSystem Specifications/Application Functions - EA4/SF045A Handwheel Angle System Arbitration)' '#SF045A_125' 'true' 'REQ:  SF045A_125' '' ; 'linktype_rmi_doors' '00012ce0 (/E-STEER Core/SubSystem Specifications/Application Functions - EA4/SF045A Handwheel Angle System Arbitration)' '#SF045A_76' 'true' 'REQ:  SF045A_76' '' } %GIDa_3946ac8c_c59b_4825_b9dc_16a7e8949749"  TreatAsAtomicUnit=on
  VrfyHwAgCorrln : Subsystem  RequirementInfo="{'linktype_rmi_doors' '00012ce0 (/E-STEER Core/SubSystem Specifications/Application Functions - EA4/SF045A Handwheel Angle System Arbitration)' '#SF045A_71' 'true' 'REQ:  SF045A_71' '' ; 'linktype_rmi_doors' '00012ce0 (/E-STEER Core/SubSystem Specifications/Application Functions - EA4/SF045A Handwheel Angle System Arbitration)' '#SF045A_73' 'true' 'REQ:  SF045A_73' '' } %GIDa_6eeb23dd_4f20_49aa_b378_2b29c2dc9482"  TreatAsAtomicUnit=on
  SrcSeln : Outport
  HwAgOut : Outport  Port=2
  HwAgConfOut : Outport  Port=3
  HwAgNotCorrd : Outport  Port=4
  wires:
  HwAgSnsrls/1 -> [HwAgSnsrls]
  [HwAgCorrdConf] -> VrfyHwAgCorrln/2(HwAgCorrdConf)
  If/2 -> SnsrlsHwAgSeln/Action
  HwAgCorrd/1 -> [HwAgCorrd]
  Merge/1 -> HwAgOut/1
  If/1 -> VrfyHwAgCorrln/Action
  [HwAgSnsrls] -> SnsrlsHwAgSeln/1(HwAgSnsrls)
  [HwAgSnsrlsConf] -> SnsrlsHwAgSeln/2(HwAgSnsrlsConf)
  [HwAgCorrd] -> VrfyHwAgCorrln/1(HwAgCorrd)
  HwAg/1 -> VrfyHwAgCorrln/3(HwAg)
  Merge2/1 -> HwAgNotCorrd/1
  Merge3/1 -> SrcSeln/1
  Merge1/1 -> HwAgConfOut/1
  HwAgSnsrlsConf/1 -> [HwAgSnsrlsConf], Relational Operator2/2
  Relational Operator2/1 -> If/1
  VrfyHwAgCorrln/1(HwAgOut) -> Merge/1
  SnsrlsHwAgSeln/1(HwAgOut) -> Merge/2
  VrfyHwAgCorrln/2(HwAgConfOut) -> Merge1/1
  SnsrlsHwAgSeln/2(HwAgConfOut) -> Merge1/2
  VrfyHwAgCorrln/3("HwAgNotCorrd ") -> Merge2/1
  SnsrlsHwAgSeln/3(HwAgNotCorrd) -> Merge2/2
  SnsrlsHwAgSeln/4(SrcSeln) -> Merge3/2
  VrfyHwAgCorrln/4(SrcSeln) -> Merge3/1
  HwAgCorrdConf/1 -> [HwAgCorrdConf], Relational Operator2/1
